simulink model "simulation"  (R2023b)
settings: Solver=VariableStepAuto  StartTime=0.0  StopTime=10.0  RelTol=1e-3
values from neighbouring files (symbols this model uses):
  a0 = 8    [script.m]
  a1 = 2    [script.m]
  b = 4    [script.m]
  du = 5    [script.m]
  t0 = 0    [script.m]
  u0 = 0    [script.m]
  x10 = initialConditions(i)    [script.m]
settings Model: Creator=igorkrzywda  LastModifiedBy=igorkrzywda

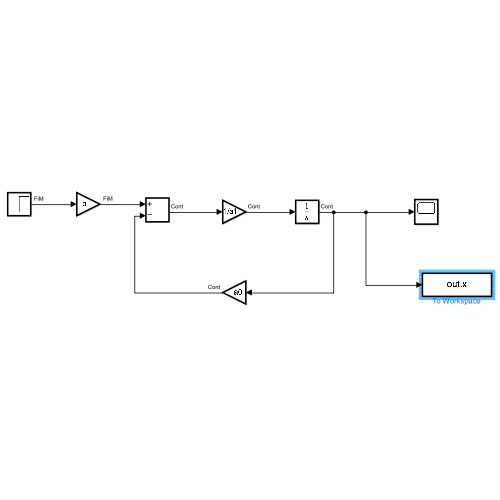
[thumbnail: Simulink's stored preview of the top-level diagram]
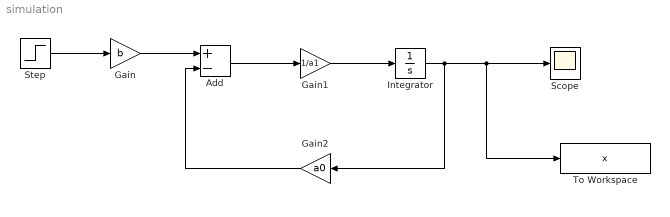
== system simulation ==
  Add : Sum  Inputs=+-
  Gain : Gain  Gain=b
  Gain1 : Gain  Gain=1/a1
  Gain2 : Gain  Gain=a0
  Integrator : Integrator  InitialCondition=x10
  Scope : Scope
  Step : Step  Time=t0  Before=u0  After=u0 + du  SampleTime=0
  To Workspace : ToWorkspace  VariableName=x  SampleTime=-1
  wires:
  Step/1 -> Gain/1
  Gain/1 -> Add/1
  Add/1 -> Gain1/1
  Gain1/1 -> Integrator/1
  Integrator/1 -> Gain2/1, To Workspace/1, Scope/1
  Gain2/1 -> Add/2
